simulink model "StraightACC_cs_old"  (R2016a)
settings: Solver=ode5  SolverMode=SingleTasking  StartTime=0.0  StopTime=10  FixedStep=1/1000  RelTol=1e-3
PreLoadFcn:
  | mbxruntime.callbacks.PreLoadFcn(bdroot);
PostLoadFcn:
  | mbxruntime.callbacks.PostLoadFcn(bdroot);
InitFcn:
  | mbxruntime.callbacks.InitFcn(bdroot);
StartFcn:
  | mbxruntime.callbacks.StartFcn(bdroot);
StopFcn:
  | mbxruntime.callbacks.StopFcn(bdroot);
model workspace (MAT data in the model file):
  mbox_table : struct (value not decoded)
  model_closed = 0
  sim_status = 0
values from neighbouring files (symbols this model uses):
  CCCDuration = 5    [PreScan_Runscript.m]
  V0 = CCCArray(2*CCCCasei-1)    [PreScan_Runscript.m]
  V1 = CCCArray(2*CCCCasei)    [PreScan_Runscript.m]
  VAccuracyIn = 0.8    [PreScan_Runscript.m]
  VDurationIn = 2    [PreScan_Runscript.m]
  VPIDIn = CCCArray(2*CCCCasei-1)    [PreScan_Runscript.m]
  VToleranceIn = 1    [PreScan_Runscript.m]
undefined symbols (not defined in the file or in its folder): ADASID, BMotor1, BMotor2, BrkDelayTime, DControlB, Delay1, Delay2, DiscIntNeverNeededParam, IControlB, JMotor1, JMotor2, PControlB, PreScanCarSimLoadFcn, ratioGearF, ratioGearR, TorqDelayTime, Tstep
undefined symbols (not defined in the file): WheelL0, WheelL1, WheelR0, WheelR1
libraries: simulink x13, simulink_extras x11, PreScanSimulinkLibrary x9, MyLib x3, Solver_SF x2, pil_lib x1, PreScanUsefulBlocks x1
(part 3 of 9)

== system StraightACC_cs_old/Roewe_550_S_Sedan_1/WheelDisplacement_Mux ==
  Steering Angle Front [rad] : Inport  Tag=inport/JointGroup  SampleTime=10/1000  BusOutputAsStruct=on
  Steering Angle Rear [rad] : Inport  Tag=inport/JointGroup  Port=2  SampleTime=10/1000  BusOutputAsStruct=on
  Rotation [rad] : Inport  Tag=inport/JointGroup  Port=3  SampleTime=10/1000  BusOutputAsStruct=on
  zDisp FL [m] : Inport  Tag=inport/JointGroup  Port=4  SampleTime=10/1000  BusOutputAsStruct=on
  zDisp FR [m] : Inport  Tag=inport/JointGroup  Port=5  SampleTime=10/1000  BusOutputAsStruct=on
  zDisp RL [m] : Inport  Tag=inport/JointGroup  Port=6  SampleTime=10/1000  BusOutputAsStruct=on
  zDisp RR [m] : Inport  Tag=inport/JointGroup  Port=7  SampleTime=10/1000  BusOutputAsStruct=on
  Ground_{1..12} (12 alike) : Ground
  WheelL0_Mux : Subsystem  Tag=mux/Joint  mask(PreScan Mux Block){DisplayName=WheelL0}
      mask prompts: DisplayName "Display Name"
      mask help:
      | This block simulates a generic joint used for generic models. This joint can be enabled/disabled from the GUI.
      |
      | For more information, please click Help.
      settings: DeleteFcn=PreScanBlockDeleteFcn;
      mask Help: eval('openHelp(254)')
  WheelL1_Mux : Subsystem  Tag=mux/Joint  mask(PreScan Mux Block){DisplayName=WheelL1}
      mask prompts: DisplayName "Display Name"
      mask help:
      | This block simulates a generic joint used for generic models. This joint can be enabled/disabled from the GUI.
      |
      | For more information, please click Help.
      settings: DeleteFcn=PreScanBlockDeleteFcn;
      mask Help: eval('openHelp(254)')
  WheelR0_Mux : Subsystem  Tag=mux/Joint  mask(PreScan Mux Block){DisplayName=WheelR0}
      mask prompts: DisplayName "Display Name"
      mask help:
      | This block simulates a generic joint used for generic models. This joint can be enabled/disabled from the GUI.
      |
      | For more information, please click Help.
      settings: DeleteFcn=PreScanBlockDeleteFcn;
      mask Help: eval('openHelp(254)')
  WheelR1_Mux : Subsystem  Tag=mux/Joint  mask(PreScan Mux Block){DisplayName=WheelR1}
      mask prompts: DisplayName "Display Name"
      mask help:
      | This block simulates a generic joint used for generic models. This joint can be enabled/disabled from the GUI.
      |
      | For more information, please click Help.
      settings: DeleteFcn=PreScanBlockDeleteFcn;
      mask Help: eval('openHelp(254)')
  WheelL0_Roewe_550_S_Sedan_1 : Outport  Tag=outport/JointActuator  OutDataTypeStr=Bus: PRESCAN_POSE_DATA  SampleTime=10/1000
  WheelL1_Roewe_550_S_Sedan_1 : Outport  Tag=outport/JointActuator  Port=2  OutDataTypeStr=Bus: PRESCAN_POSE_DATA  SampleTime=10/1000
  WheelR0_Roewe_550_S_Sedan_1 : Outport  Tag=outport/JointActuator  Port=3  OutDataTypeStr=Bus: PRESCAN_POSE_DATA  SampleTime=10/1000
  WheelR1_Roewe_550_S_Sedan_1 : Outport  Tag=outport/JointActuator  Port=4  OutDataTypeStr=Bus: PRESCAN_POSE_DATA  SampleTime=10/1000
  wires:
  WheelL0_Mux/1(Joint) -> WheelL0_Roewe_550_S_Sedan_1/1
  WheelL1_Mux/1(Joint) -> WheelL1_Roewe_550_S_Sedan_1/1
  WheelR0_Mux/1(Joint) -> WheelR0_Roewe_550_S_Sedan_1/1
  WheelR1_Mux/1(Joint) -> WheelR1_Roewe_550_S_Sedan_1/1
  Steering Angle Front [rad]/1 -> WheelR0_Mux/6(Yaw [rad]), WheelL0_Mux/6(Yaw [rad])
  Steering Angle Rear [rad]/1 -> WheelR1_Mux/6(Yaw [rad]), WheelL1_Mux/6(Yaw [rad])
  Rotation [rad]/1 -> WheelR0_Mux/5(Pitch [rad]), WheelL0_Mux/5(Pitch [rad]), WheelR1_Mux/5(Pitch [rad]), WheelL1_Mux/5(Pitch [rad])
  zDisp FL [m]/1 -> WheelL0_Mux/3(Z [m])
  zDisp FR [m]/1 -> WheelR0_Mux/3(Z [m])
  zDisp RL [m]/1 -> WheelL1_Mux/3(Z [m])
  zDisp RR [m]/1 -> WheelR1_Mux/3(Z [m])
  Ground_1/1 -> WheelL0_Mux/1(X [m])
  Ground_2/1 -> WheelL0_Mux/2(Y [m])
  Ground_3/1 -> WheelL0_Mux/4(Roll [rad])
  Ground_4/1 -> WheelL1_Mux/1(X [m])
  Ground_5/1 -> WheelL1_Mux/2(Y [m])
  Ground_6/1 -> WheelL1_Mux/4(Roll [rad])
  Ground_7/1 -> WheelR0_Mux/1(X [m])
  Ground_8/1 -> WheelR0_Mux/2(Y [m])
  Ground_9/1 -> WheelR0_Mux/4(Roll [rad])
  Ground_10/1 -> WheelR1_Mux/1(X [m])
  Ground_11/1 -> WheelR1_Mux/2(Y [m])
  Ground_12/1 -> WheelR1_Mux/4(Roll [rad])

== system StraightACC_cs_old/WheelL0_Roewe_550_S_Sedan_1/Actuator ==
  Joint : Inport
  Bus Selector : BusSelector  OutputSignals=POSITION,ORIENTATION
  visu_Rotate : Subsystem  mask(RPYActuator){UniqueID=UniqueID, Object3DID=Rotate_ObjectID3D, TimeStep=TimeStep}
      mask prompts: UniqueID "Auto-Assigned: Unique ID"; Object3DID "Auto-Assigned: Child 3D Object ID"; TimeStep "Auto-Assigned: Upload Period [s]"
      mask help: Applies angles update to selected child object
      mask Help:
      | Applies position update to selected child object
      | 
      | - UniqueID (double)   : Unique ID of the parent actor
      | - Object3DID (string) : Name of the child 3D object
      mask Display: port_label('input', 1, ['visu_Rotate_' Object3DID])
  visu_Translate : Subsystem  mask(PositionActuator){UniqueID=UniqueID, Object3DID=Translate_ObjectID3D, TimeStep=TimeStep}
      mask prompts: UniqueID "Auto-Assigned: Unique ID"; Object3DID "Auto-Assigned: Child 3D Object ID"; TimeStep "Auto-Assigned: Upload Period [s]"
      mask help: Applies position update to selected child object
      mask Help:
      | Applies position update to selected child object
      | 
      | - UniqueID (double)   : Unique ID of the parent actor
      | - Object3DID (string) : Name of the child 3D object
      mask Display: port_label('input', 1, ['visu_Translate_' Object3DID])
  wires:
  Bus Selector/2 -> visu_Rotate/1(In1)  "<ORIENTATION>"
  Bus Selector/1 -> visu_Translate/1(In1)  "<POSITION>"
  Joint/1 -> Bus Selector/1

== system StraightACC_cs_old/WheelL1_Roewe_550_S_Sedan_1/Actuator ==
  Joint : Inport
  Bus Selector : BusSelector  OutputSignals=POSITION,ORIENTATION
  visu_Rotate : Subsystem  mask(RPYActuator){UniqueID=UniqueID, Object3DID=Rotate_ObjectID3D, TimeStep=TimeStep}
      mask prompts: UniqueID "Auto-Assigned: Unique ID"; Object3DID "Auto-Assigned: Child 3D Object ID"; TimeStep "Auto-Assigned: Upload Period [s]"
      mask help: Applies angles update to selected child object
      mask Help:
      | Applies position update to selected child object
      | 
      | - UniqueID (double)   : Unique ID of the parent actor
      | - Object3DID (string) : Name of the child 3D object
      mask Display: port_label('input', 1, ['visu_Rotate_' Object3DID])
  visu_Translate : Subsystem  mask(PositionActuator){UniqueID=UniqueID, Object3DID=Translate_ObjectID3D, TimeStep=TimeStep}
      mask prompts: UniqueID "Auto-Assigned: Unique ID"; Object3DID "Auto-Assigned: Child 3D Object ID"; TimeStep "Auto-Assigned: Upload Period [s]"
      mask help: Applies position update to selected child object
      mask Help:
      | Applies position update to selected child object
      | 
      | - UniqueID (double)   : Unique ID of the parent actor
      | - Object3DID (string) : Name of the child 3D object
      mask Display: port_label('input', 1, ['visu_Translate_' Object3DID])
  wires:
  Bus Selector/2 -> visu_Rotate/1(In1)  "<ORIENTATION>"
  Bus Selector/1 -> visu_Translate/1(In1)  "<POSITION>"
  Joint/1 -> Bus Selector/1

== system StraightACC_cs_old/WheelR0_Roewe_550_S_Sedan_1/Actuator ==
  Joint : Inport
  Bus Selector : BusSelector  OutputSignals=POSITION,ORIENTATION
  visu_Rotate : Subsystem  mask(RPYActuator){UniqueID=UniqueID, Object3DID=Rotate_ObjectID3D, TimeStep=TimeStep}
      mask prompts: UniqueID "Auto-Assigned: Unique ID"; Object3DID "Auto-Assigned: Child 3D Object ID"; TimeStep "Auto-Assigned: Upload Period [s]"
      mask help: Applies angles update to selected child object
      mask Help:
      | Applies position update to selected child object
      | 
      | - UniqueID (double)   : Unique ID of the parent actor
      | - Object3DID (string) : Name of the child 3D object
      mask Display: port_label('input', 1, ['visu_Rotate_' Object3DID])
  visu_Translate : Subsystem  mask(PositionActuator){UniqueID=UniqueID, Object3DID=Translate_ObjectID3D, TimeStep=TimeStep}
      mask prompts: UniqueID "Auto-Assigned: Unique ID"; Object3DID "Auto-Assigned: Child 3D Object ID"; TimeStep "Auto-Assigned: Upload Period [s]"
      mask help: Applies position update to selected child object
      mask Help:
      | Applies position update to selected child object
      | 
      | - UniqueID (double)   : Unique ID of the parent actor
      | - Object3DID (string) : Name of the child 3D object
      mask Display: port_label('input', 1, ['visu_Translate_' Object3DID])
  wires:
  Bus Selector/2 -> visu_Rotate/1(In1)  "<ORIENTATION>"
  Bus Selector/1 -> visu_Translate/1(In1)  "<POSITION>"
  Joint/1 -> Bus Selector/1

== system StraightACC_cs_old/WheelR1_Roewe_550_S_Sedan_1/Actuator ==
  Joint : Inport
  Bus Selector : BusSelector  OutputSignals=POSITION,ORIENTATION
  visu_Rotate : Subsystem  mask(RPYActuator){UniqueID=UniqueID, Object3DID=Rotate_ObjectID3D, TimeStep=TimeStep}
      mask prompts: UniqueID "Auto-Assigned: Unique ID"; Object3DID "Auto-Assigned: Child 3D Object ID"; TimeStep "Auto-Assigned: Upload Period [s]"
      mask help: Applies angles update to selected child object
      mask Help:
      | Applies position update to selected child object
      | 
      | - UniqueID (double)   : Unique ID of the parent actor
      | - Object3DID (string) : Name of the child 3D object
      mask Display: port_label('input', 1, ['visu_Rotate_' Object3DID])
  visu_Translate : Subsystem  mask(PositionActuator){UniqueID=UniqueID, Object3DID=Translate_ObjectID3D, TimeStep=TimeStep}
      mask prompts: UniqueID "Auto-Assigned: Unique ID"; Object3DID "Auto-Assigned: Child 3D Object ID"; TimeStep "Auto-Assigned: Upload Period [s]"
      mask help: Applies position update to selected child object
      mask Help:
      | Applies position update to selected child object
      | 
      | - UniqueID (double)   : Unique ID of the parent actor
      | - Object3DID (string) : Name of the child 3D object
      mask Display: port_label('input', 1, ['visu_Translate_' Object3DID])
  wires:
  Bus Selector/2 -> visu_Rotate/1(In1)  "<ORIENTATION>"
  Bus Selector/1 -> visu_Translate/1(In1)  "<POSITION>"
  Joint/1 -> Bus Selector/1

== system StraightACC_cs_old/Audi_A8_Sedan_1/SELF_Demux/compas converter ==
  rotz [rad] : Inport
  cart2compas : Subsystem
  rad2deg : Gain  Gain=180/pi
  heading [deg] : Outport
  wires:
  rad2deg/1 -> cart2compas/1(Angle [deg])
  rotz [rad]/1 -> rad2deg/1
  cart2compas/1(heading [deg]) -> heading [deg]/1

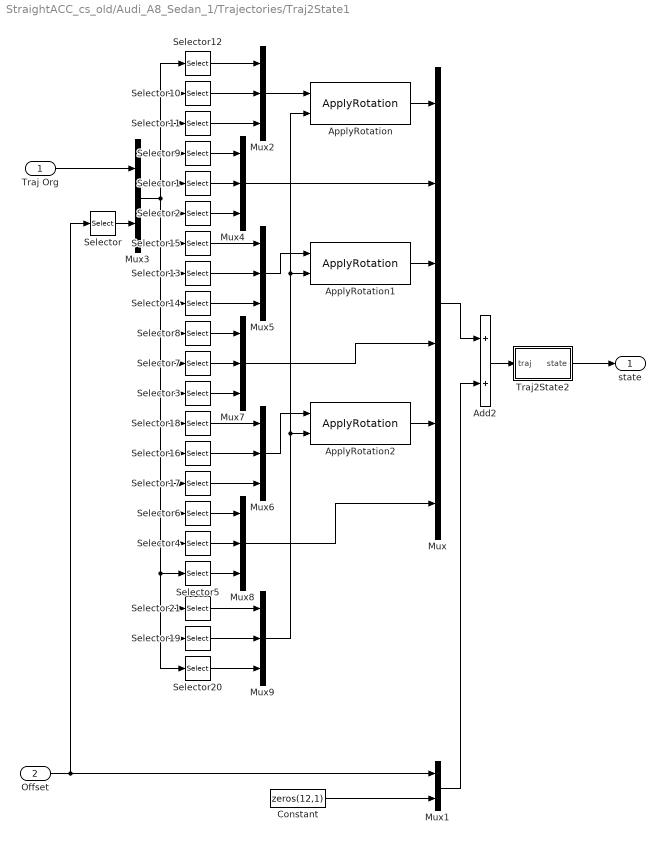
== system StraightACC_cs_old/Audi_A8_Sedan_1/Trajectories/Traj2State1 ==
  Traj Org : Inport
  Offset : Inport  Port=2
  Add2 : Sum
  ApplyRotation : PreScanSimulinkLibrary/ApplyRotation
  ApplyRotation1 : PreScanSimulinkLibrary/ApplyRotation
  ApplyRotation2 : PreScanSimulinkLibrary/ApplyRotation
  Constant : Constant  Value=zeros(12,1)
  Mux : Mux  Inputs=6
  Mux1 : Mux  Inputs=2
  Mux{2,4..9} (7 alike) : Mux  Inputs=3
  Mux3 : Mux  Inputs=2
  Selector : Selector  InputPortWidth=6  IndexOptions=Index vector (dialog)  Indices=[4 5 6]  OutputSizes=1
  Selector1 : Selector  InputPortWidth=21  IndexOptions=Index vector (dialog)  Indices=[5]  OutputSizes=1
  Selector10 : Selector  InputPortWidth=21  IndexOptions=Index vector (dialog)  Indices=[2]  OutputSizes=1
  Selector11 : Selector  InputPortWidth=21  IndexOptions=Index vector (dialog)  Indices=[3]  OutputSizes=1
  Selector12 : Selector  InputPortWidth=21  IndexOptions=Index vector (dialog)  Indices=[1]  OutputSizes=1
  Selector13 : Selector  InputPortWidth=21  IndexOptions=Index vector (dialog)  Indices=[8]  OutputSizes=1
  Selector14 : Selector  InputPortWidth=21  IndexOptions=Index vector (dialog)  Indices=[9]  OutputSizes=1
  Selector15 : Selector  InputPortWidth=21  IndexOptions=Index vector (dialog)  Indices=[7]  OutputSizes=1
  Selector16 : Selector  InputPortWidth=21  IndexOptions=Index vector (dialog)  Indices=[14]  OutputSizes=1
  Selector17 : Selector  InputPortWidth=21  IndexOptions=Index vector (dialog)  Indices=[15]  OutputSizes=1
  Selector18 : Selector  InputPortWidth=21  IndexOptions=Index vector (dialog)  Indices=[13]  OutputSizes=1
  Selector19 : Selector  InputPortWidth=21  IndexOptions=Index vector (dialog)  Indices=[20]  OutputSizes=1
  Selector2 : Selector  InputPortWidth=21  IndexOptions=Index vector (dialog)  Indices=[6]  OutputSizes=1
  Selector20 : Selector  InputPortWidth=21  IndexOptions=Index vector (dialog)  Indices=[21]  OutputSizes=1
  Selector21 : Selector  InputPortWidth=21  IndexOptions=Index vector (dialog)  Indices=[19]  OutputSizes=1
  Selector3 : Selector  InputPortWidth=21  IndexOptions=Index vector (dialog)  Indices=[12]  OutputSizes=1
  Selector4 : Selector  InputPortWidth=21  IndexOptions=Index vector (dialog)  Indices=[17]  OutputSizes=1
  Selector5 : Selector  InputPortWidth=21  IndexOptions=Index vector (dialog)  Indices=[18]  OutputSizes=1
  Selector6 : Selector  InputPortWidth=21  IndexOptions=Index vector (dialog)  Indices=[16]  OutputSizes=1
  Selector7 : Selector  InputPortWidth=21  IndexOptions=Index vector (dialog)  Indices=[11]  OutputSizes=1
  Selector8 : Selector  InputPortWidth=21  IndexOptions=Index vector (dialog)  Indices=[10]  OutputSizes=1
  Selector9 : Selector  InputPortWidth=21  IndexOptions=Index vector (dialog)  Indices=[4]  OutputSizes=1
  Traj2State2 : Subsystem
  state : Outport
  wires:
  Mux9/1 -> ApplyRotation2/2, ApplyRotation1/2, ApplyRotation/2
  Selector20/1 -> Mux9/3
  Selector19/1 -> Mux9/2
  Selector21/1 -> Mux9/1
  Selector5/1 -> Mux8/3
  Selector4/1 -> Mux8/2
  Selector6/1 -> Mux8/1
  Mux8/1 -> Mux/6
  Mux6/1 -> ApplyRotation2/1
  Mux7/1 -> Mux/4
  ApplyRotation2/1 -> Mux/5
  Selector3/1 -> Mux7/3
  Selector7/1 -> Mux7/2
  Selector8/1 -> Mux7/1
  Mux4/1 -> Mux/2
  Mux5/1 -> ApplyRotation1/1
  ApplyRotation1/1 -> Mux/3
  Mux2/1 -> ApplyRotation/1
  ApplyRotation/1 -> Mux/1
  Selector2/1 -> Mux4/3
  Selector1/1 -> Mux4/2
  Selector9/1 -> Mux4/1
  Selector17/1 -> Mux6/3
  Selector16/1 -> Mux6/2
  Selector18/1 -> Mux6/1
  Selector14/1 -> Mux5/3
  Selector13/1 -> Mux5/2
  Selector15/1 -> Mux5/1
  Selector11/1 -> Mux2/3
  Selector10/1 -> Mux2/2
  Selector12/1 -> Mux2/1
  Mux3/1 -> Selector8/1, Selector7/1, Selector3/1, Selector18/1, Selector16/1, Selector17/1, Selector6/1, Selector20/1, Selector19/1, Selector21/1, Selector5/1, Selector4/1, Selector14/1, Selector13/1, Selector15/1, Selector2/1, Selector1/1, Selector9/1, Selector12/1, Selector10/1, Selector11/1
  Mux1/1 -> Add2/2
  Constant/1 -> Mux1/2
  Add2/1 -> Traj2State2/1(traj)
  Selector/1 -> Mux3/2
  Traj Org/1 -> Mux3/1
  Offset/1 -> Mux1/1, Selector/1
  Mux/1 -> Add2/1
  Traj2State2/1(state) -> state/1

== system StraightACC_cs_old/Audi_A8_Sedan_1/Trajectories/TrajCoGOffset ==
  State In : Inport
  Add : Sum  Inputs=+-+
  Add1 : Sum
  ApplyRotation : PreScanSimulinkLibrary/ApplyRotation
  ApplyRotation1 : PreScanSimulinkLibrary/ApplyRotation
  CoG Offset : Constant  Value=[0 0 CoGOffsetZ]
  Degrees to Radians : simulink_extras/Transformations/Degrees to Radians
  Demux1 : Demux  Outputs=[3 3 3]
  Mux : Mux  Inputs=[3 3 3]
  Orientation : Constant  Value=[InitRoll InitPitch 0]
  State Out : Outport
  wires:
  State In/1 -> Demux1/1
  Demux1/1 -> Add/1
  Add/1 -> Mux/1
  Demux1/3 -> Mux/3, Add1/2
  Mux/1 -> State Out/1
  Demux1/2 -> Mux/2
  Orientation/1 -> Degrees to Radians/1
  ApplyRotation/1 -> Add/3
  ApplyRotation1/1 -> Add/2
  Add1/1 -> ApplyRotation/2
  CoG Offset/1 -> ApplyRotation1/1, ApplyRotation/1
  Degrees to Radians/1 -> Add1/1, ApplyRotation1/2

== system StraightACC_cs_old/Audi_A8_Sedan_1/Trajectories/Trajectory_1 ==
  From Workspace : FromWorkspace  VariableName=trajectory  SampleTime=TimeStep  OutputAfterFinalValue=Holding final value
  From Workspace1 : FromWorkspace  VariableName=trajectory  SampleTime=TimeStep  OutputAfterFinalValue=Setting to zero
  Mux : Mux  Inputs=2
  Selector1 : Selector  InputPortWidth=24  IndexOptions=Index vector (dialog)  Indices=[7:18]  OutputSizes=1
  Selector9 : Selector  InputPortWidth=24  IndexOptions=Index vector (dialog)  Indices=[1:6]  OutputSizes=1
  trajectory : Outport
  wires:
  From Workspace/1 -> Selector9/1
  From Workspace1/1 -> Selector1/1
  Mux/1 -> trajectory/1
  Selector9/1 -> Mux/1
  Selector1/1 -> Mux/2

== system StraightACC_cs_old/Roewe_550_S_Sedan_1/CarSim I//O/ACCAEB ==
  ACCAEBIn : Inport  OutDataTypeStr=Bus: AccAebInputs  BusOutputAsStruct=on
  ACCAEB_sfcn : pil_lib/PIL Block  SimulationMode=SIL  IsTopModelPIL=off  CodeDir=D:\Temp\SimCodeGen\Dest\ACCAEB_ert_rtw  ConfigName=Software-in-the-Loop (SIL)
  __InputSSForSFun__ : Subsystem
  __OutputSSForSFun__ : Subsystem
  ACCAEBOut : Outport
  wires:
  ACCAEBIn/1 -> __InputSSForSFun__/1(ACCAEBIn)
  __InputSSForSFun__/1(__UniqueOutportName__1__) -> ACCAEB_sfcn/1
  ACCAEB_sfcn/1 -> __OutputSSForSFun__/1(__UniqueInportName__1__)
  ACCAEB_sfcn/2 -> __OutputSSForSFun__/2(__UniqueInportName__2__)
  ACCAEB_sfcn/3 -> __OutputSSForSFun__/3(__UniqueInportName__3__)
  ACCAEB_sfcn/4 -> __OutputSSForSFun__/4(__UniqueInportName__4__)
  ACCAEB_sfcn/5 -> __OutputSSForSFun__/5(__UniqueInportName__5__)
  ACCAEB_sfcn/6 -> __OutputSSForSFun__/6(__UniqueInportName__6__)
  ACCAEB_sfcn/7 -> __OutputSSForSFun__/7(__UniqueInportName__7__)
  ACCAEB_sfcn/8 -> __OutputSSForSFun__/8(__UniqueInportName__8__)
  ACCAEB_sfcn/9 -> __OutputSSForSFun__/9(__UniqueInportName__9__)
  ACCAEB_sfcn/10 -> __OutputSSForSFun__/10(__UniqueInportName__10__)
  ACCAEB_sfcn/11 -> __OutputSSForSFun__/11(__UniqueInportName__11__)
  ACCAEB_sfcn/12 -> __OutputSSForSFun__/12(__UniqueInportName__12__)
  ACCAEB_sfcn/13 -> __OutputSSForSFun__/13(__UniqueInportName__13__)
  ACCAEB_sfcn/14 -> __OutputSSForSFun__/14(__UniqueInportName__14__)
  ACCAEB_sfcn/15 -> __OutputSSForSFun__/15(__UniqueInportName__15__)
  ACCAEB_sfcn/16 -> __OutputSSForSFun__/16(__UniqueInportName__16__)
  ACCAEB_sfcn/17 -> __OutputSSForSFun__/17(__UniqueInportName__17__)
  ACCAEB_sfcn/18 -> __OutputSSForSFun__/18(__UniqueInportName__18__)
  ACCAEB_sfcn/19 -> __OutputSSForSFun__/19(__UniqueInportName__19__)
  ACCAEB_sfcn/20 -> __OutputSSForSFun__/20(__UniqueInportName__20__)
  ACCAEB_sfcn/21 -> __OutputSSForSFun__/21(__UniqueInportName__21__)
  ACCAEB_sfcn/22 -> __OutputSSForSFun__/22(__UniqueInportName__22__)
  ACCAEB_sfcn/23 -> __OutputSSForSFun__/23(__UniqueInportName__23__)
  ACCAEB_sfcn/24 -> __OutputSSForSFun__/24(__UniqueInportName__24__)
  ACCAEB_sfcn/25 -> __OutputSSForSFun__/25(__UniqueInportName__25__)
  ACCAEB_sfcn/26 -> __OutputSSForSFun__/26(__UniqueInportName__26__)
  ACCAEB_sfcn/27 -> __OutputSSForSFun__/27(__UniqueInportName__27__)
  ACCAEB_sfcn/28 -> __OutputSSForSFun__/28(__UniqueInportName__28__)
  ACCAEB_sfcn/29 -> __OutputSSForSFun__/29(__UniqueInportName__29__)
  ACCAEB_sfcn/30 -> __OutputSSForSFun__/30(__UniqueInportName__30__)
  ACCAEB_sfcn/31 -> __OutputSSForSFun__/31(__UniqueInportName__31__)
  ACCAEB_sfcn/32 -> __OutputSSForSFun__/32(__UniqueInportName__32__)
  ACCAEB_sfcn/33 -> __OutputSSForSFun__/33(__UniqueInportName__33__)
  ACCAEB_sfcn/34 -> __OutputSSForSFun__/34(__UniqueInportName__34__)
  ACCAEB_sfcn/35 -> __OutputSSForSFun__/35(__UniqueInportName__35__)
  ACCAEB_sfcn/36 -> __OutputSSForSFun__/36(__UniqueInportName__36__)
  ACCAEB_sfcn/37 -> __OutputSSForSFun__/37(__UniqueInportName__37__)
  ACCAEB_sfcn/38 -> __OutputSSForSFun__/38(__UniqueInportName__38__)
  ACCAEB_sfcn/39 -> __OutputSSForSFun__/39(__UniqueInportName__39__)
  ACCAEB_sfcn/40 -> __OutputSSForSFun__/40(__UniqueInportName__40__)
  ACCAEB_sfcn/41 -> __OutputSSForSFun__/41(__UniqueInportName__41__)
  ACCAEB_sfcn/42 -> __OutputSSForSFun__/42(__UniqueInportName__42__)
  ACCAEB_sfcn/43 -> __OutputSSForSFun__/43(__UniqueInportName__43__)
  ACCAEB_sfcn/44 -> __OutputSSForSFun__/44(__UniqueInportName__44__)
  ACCAEB_sfcn/45 -> __OutputSSForSFun__/45(__UniqueInportName__45__)
  ACCAEB_sfcn/46 -> __OutputSSForSFun__/46(__UniqueInportName__46__)
  ACCAEB_sfcn/47 -> __OutputSSForSFun__/47(__UniqueInportName__47__)
  ACCAEB_sfcn/48 -> __OutputSSForSFun__/48(__UniqueInportName__48__)
  ACCAEB_sfcn/49 -> __OutputSSForSFun__/49(__UniqueInportName__49__)
  ACCAEB_sfcn/50 -> __OutputSSForSFun__/50(__UniqueInportName__50__)
  ACCAEB_sfcn/51 -> __OutputSSForSFun__/51(__UniqueInportName__51__)
  ACCAEB_sfcn/52 -> __OutputSSForSFun__/52(__UniqueInportName__52__)
  ACCAEB_sfcn/53 -> __OutputSSForSFun__/53(__UniqueInportName__53__)
  ACCAEB_sfcn/54 -> __OutputSSForSFun__/54(__UniqueInportName__54__)
  ACCAEB_sfcn/55 -> __OutputSSForSFun__/55(__UniqueInportName__55__)
  ACCAEB_sfcn/56 -> __OutputSSForSFun__/56(__UniqueInportName__56__)
  ACCAEB_sfcn/57 -> __OutputSSForSFun__/57(__UniqueInportName__57__)
  ACCAEB_sfcn/58 -> __OutputSSForSFun__/58(__UniqueInportName__58__)
  ACCAEB_sfcn/59 -> __OutputSSForSFun__/59(__UniqueInportName__59__)
  ACCAEB_sfcn/60 -> __OutputSSForSFun__/60(__UniqueInportName__60__)
  ACCAEB_sfcn/61 -> __OutputSSForSFun__/61(__UniqueInportName__61__)
  ACCAEB_sfcn/62 -> __OutputSSForSFun__/62(__UniqueInportName__62__)
  ACCAEB_sfcn/63 -> __OutputSSForSFun__/63(__UniqueInportName__63__)
  ACCAEB_sfcn/64 -> __OutputSSForSFun__/64(__UniqueInportName__64__)
  ACCAEB_sfcn/65 -> __OutputSSForSFun__/65(__UniqueInportName__65__)
  ACCAEB_sfcn/66 -> __OutputSSForSFun__/66(__UniqueInportName__66__)
  ACCAEB_sfcn/67 -> __OutputSSForSFun__/67(__UniqueInportName__67__)
  ACCAEB_sfcn/68 -> __OutputSSForSFun__/68(__UniqueInportName__68__)
  ACCAEB_sfcn/69 -> __OutputSSForSFun__/69(__UniqueInportName__69__)
  ACCAEB_sfcn/70 -> __OutputSSForSFun__/70(__UniqueInportName__70__)
  ACCAEB_sfcn/71 -> __OutputSSForSFun__/71(__UniqueInportName__71__)
  ACCAEB_sfcn/72 -> __OutputSSForSFun__/72(__UniqueInportName__72__)
  ACCAEB_sfcn/73 -> __OutputSSForSFun__/73(__UniqueInportName__73__)
  ACCAEB_sfcn/74 -> __OutputSSForSFun__/74(__UniqueInportName__74__)
  ACCAEB_sfcn/75 -> __OutputSSForSFun__/75(__UniqueInportName__75__)
  ACCAEB_sfcn/76 -> __OutputSSForSFun__/76(__UniqueInportName__76__)
  ACCAEB_sfcn/77 -> __OutputSSForSFun__/77(__UniqueInportName__77__)
  ACCAEB_sfcn/78 -> __OutputSSForSFun__/78(__UniqueInportName__78__)
  ACCAEB_sfcn/79 -> __OutputSSForSFun__/79(__UniqueInportName__79__)
  ACCAEB_sfcn/80 -> __OutputSSForSFun__/80(__UniqueInportName__80__)
  ACCAEB_sfcn/81 -> __OutputSSForSFun__/81(__UniqueInportName__81__)
  ACCAEB_sfcn/82 -> __OutputSSForSFun__/82(__UniqueInportName__82__)
  ACCAEB_sfcn/83 -> __OutputSSForSFun__/83(__UniqueInportName__83__)
  ACCAEB_sfcn/84 -> __OutputSSForSFun__/84(__UniqueInportName__84__)
  ACCAEB_sfcn/85 -> __OutputSSForSFun__/85(__UniqueInportName__85__)
  ACCAEB_sfcn/86 -> __OutputSSForSFun__/86(__UniqueInportName__86__)
  ACCAEB_sfcn/87 -> __OutputSSForSFun__/87(__UniqueInportName__87__)
  ACCAEB_sfcn/88 -> __OutputSSForSFun__/88(__UniqueInportName__88__)
  ACCAEB_sfcn/89 -> __OutputSSForSFun__/89(__UniqueInportName__89__)
  ACCAEB_sfcn/90 -> __OutputSSForSFun__/90(__UniqueInportName__90__)
  ACCAEB_sfcn/91 -> __OutputSSForSFun__/91(__UniqueInportName__91__)
  ACCAEB_sfcn/92 -> __OutputSSForSFun__/92(__UniqueInportName__92__)
  ACCAEB_sfcn/93 -> __OutputSSForSFun__/93(__UniqueInportName__93__)
  ACCAEB_sfcn/94 -> __OutputSSForSFun__/94(__UniqueInportName__94__)
  ACCAEB_sfcn/95 -> __OutputSSForSFun__/95(__UniqueInportName__95__)
  ACCAEB_sfcn/96 -> __OutputSSForSFun__/96(__UniqueInportName__96__)
  ACCAEB_sfcn/97 -> __OutputSSForSFun__/97(__UniqueInportName__97__)
  ACCAEB_sfcn/98 -> __OutputSSForSFun__/98(__UniqueInportName__98__)
  __OutputSSForSFun__/1(ACCAEBOut) -> ACCAEBOut/1

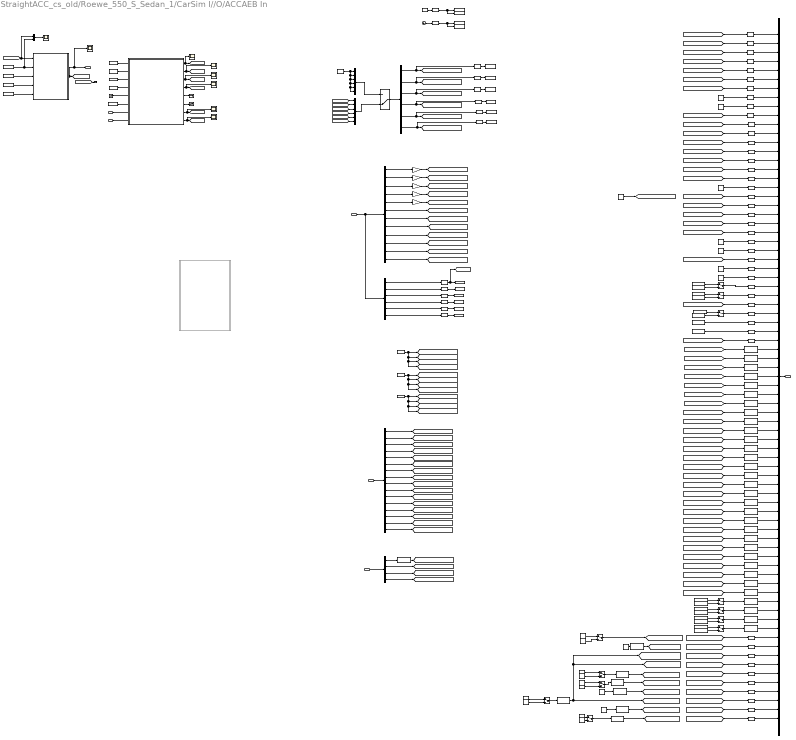
== system StraightACC_cs_old/Roewe_550_S_Sedan_1/CarSim I//O/ACCAEB In ==
  note: Here was constant 1, dont know why
  CarSimOut : Inport
  LanesInfo : Inport  Port=2
  FRadarOut : Inport  Port=3
  SetSpd : Inport  Port=4
  MemSpd : Inport  Port=5
  BrkPdlPos_H1HSC1_d1 : Constant  Value=0  OutDataTypeStr=double
  BrkPdlPos_H1HSC1_d2 : Constant  Value=0  OutDataTypeStr=uint8
  Bus Creator1 : BusCreator  Inputs=77
  Bus Selector : BusSelector  OutputSignals=Lane1C0,Lane1C1,Lane1C2,Lane1C3,Lane2C0,Lane2C1,Lane2C2,Lane2C3,Lane3C0,Lane3C1,Lane3C2,Lane3C3,Lane4C0,Lane4C1,Lane4C2,Lane4C3
  Bus Selector1 : BusSelector  OutputSignals=WhlGndVelRDrvn_H1HSC2_d[km/h] (signal 38),WhlGndVelLDrvn_H1HSC2_d[km/h] (signal 39),WhlGndVelRNonDrvn_H1HSC2_d[km/h] (signal 40),WhlGndVelLNonDrvn_H1HSC2_d[km/h] (signal 41),VSELongtAcc_H1HSC1_d[g] (signal 42),VehDynYawRate_H1HSC1_d[deg/s] (signal 43),EnSpdHSC1_d[rpm] (signal 36),SteeringWheelAngle[deg] (signal 34),StrgWhlAngGrd_HSC2_d[deg/s] (signal 44),EnToqActuExtdRngHSC1_d[N M] (signal 37),AccelEfctvPosHSC1_d (signal 46),AccelActuPosHSC1_d (signal 45)
  Bus Selector2 : BusSelector  OutputSignals=IDLockOn,Y_LockOn,X_LockOn,Vx_LockOn
  Bus Selector3 : BusSelector  OutputSignals=VehicleCoG_Vx[km/h] (signal 4),SteeringWheelAngle[deg] (signal 34),Ax_SM[g] (signal 54),Ay_SM[g] (signal 55),VehDynYawRate_H1HSC1_d[deg/s] (signal 43),StrgWhlAngGrd_HSC2_d[deg/s] (signal 44)
  CanclSW : Scope
  Chart : Stateflow chart  TreatAsAtomicUnit=on
  Clock1 : Clock
  Constant : Constant  Value=2
  Constant{1,5,13,93,102,104..105,107,110..111} (10 alike) : Constant  Value=0
  Constant{7,94,103,106,108..109,112..113} (8 alike) : Constant
  Constant15 : Constant  Value=VPIDIn
  Constant16 : Constant  Value=VToleranceIn
  Constant17 : Constant  Value=VAccuracyIn
  Constant18 : Constant  Value=VDurationIn
  Constant19 : Constant  Value=ADASID
  Constant2 : Constant  Value=95
  Constant20 : Constant  Value=V0
  Constant21 : Constant  Value=V1
  Constant3 : Constant  Value=1199
  Constant4 : Constant  Value=-848
  Constant6 : Constant  Value=CCCDuration
  DA_IN_DgrObjSyncCtr_u1 : Constant  Value=0  OutDataTypeStr=uint8
  DA_IN_DgrObjSyncCtr_u2 : Constant  Value=0  OutDataTypeStr=uint8
  DA_IN_DgrObjSyncCtr_u3 : Constant  Value=0  OutDataTypeStr=uint8
  Data Type Conversion{,1,4..8,10..12,23,28..29,31..32,45,58,66,73,86,89,115,120,124} (24 alike) : DataTypeConversion  OutDataTypeStr=uint8
  Data Type Conversion{2..3,13..22,24..27,30,35..40,84..85,92..94,116,126..129} (33 alike) : DataTypeConversion  OutDataTypeStr=double
  Data Type Conversion{9,87..88,90..91,117..119,121..123,125} (12 alike) : DataTypeConversion  OutDataTypeStr=single
  Data Type Conversion{33..34,80..83} (6 alike) : DataTypeConversion  OutDataTypeStr=boolean
  Data Type Conversion{46..48,55..57,60..65,67..72,74..79} (24 alike) : DataTypeConversion
  Demux : Demux  Outputs=6
  DrvrSbltAtcHSC1_u1 : Constant  OutDataTypeStr=uint8
  EPBAppcnStsHSC1_u1 : Constant  Value=0  OutDataTypeStr=uint8
  EnTypHSC2_u1 : Constant  OutDataTypeStr=uint8
  FntLatDist10 : Constant  Value=0  OutDataTypeStr=double
      settings: AttributesFormatString=%<OutDataTypeStr>
  FntLatDist11 : Constant  Value=13  OutDataTypeStr=double
      settings: AttributesFormatString=%<OutDataTypeStr>
  FntLatDist12 : Constant  Value=0  OutDataTypeStr=double
      settings: AttributesFormatString=%<OutDataTypeStr>
  FntLatDist7 : Constant  Value=3  OutDataTypeStr=double
      settings: AttributesFormatString=%<OutDataTypeStr>
  FntLatDist8 : Constant  Value=0  OutDataTypeStr=double
      settings: AttributesFormatString=%<OutDataTypeStr>
  FntLatDist9 : Constant  OutDataTypeStr=double
      settings: AttributesFormatString=%<OutDataTypeStr>
  Gain{,1..3} (4 alike) : Gain  Gain=1/3.6
  Gain4 : Gain  Gain=9.8
  Ground4 : Ground
  ID_LOCKON_u5 : Constant  Value=5  OutDataTypeStr=uint8
  ID_LOCKON_u6 : Constant  Value=0  OutDataTypeStr=uint8
  ID_LOCKON_u7 : Constant  Value=5  OutDataTypeStr=uint8
  ID_LOCKON_u9 : Constant  Value=0  OutDataTypeStr=uint8
  MATLAB Function : MATLAB Function  Commented=on  TreatAsAtomicUnit=on
  Manual Switch : ManualSwitch  CurrentSetting=0
  Manual Switch{56,60..70} (12 alike) : ManualSwitch
  Mux : Mux  Inputs=6
  Mux1 : Mux  Inputs=6
  Mux2 : Mux  Inputs=2
  OnSW : Scope
  RsmSW : Scope
  SetSW : Scope
  SpdDecSW : Scope
  SpdIncSW : Scope
  Steady? : Scope
  SysPwrMd_H1HSC1_u1 : Constant  Value=3  OutDataTypeStr=uint8
      settings: AttributesFormatString=%<DataType=%<OutDataTypeStr>>
  Terminator4 : Terminator
  Terminator5 : Terminator
  Terminator_1 : Terminator
  To Workspace : ToWorkspace  VariableName=SpdIncSw  SampleTime=-1
  To Workspace1 : ToWorkspace  VariableName=SpdDecSw  SampleTime=-1
  To Workspace10 : ToWorkspace  VariableName=Vx  SampleTime=-1
  To Workspace11 : ToWorkspace  VariableName=AVz  SampleTime=-1
  To Workspace12 : ToWorkspace  VariableName=Steer_SW  SampleTime=-1
  To Workspace13 : ToWorkspace  VariableName=StrAV_SW  SampleTime=-1
  To Workspace14 : ToWorkspace  VariableName=Time  SampleTime=-1
  To Workspace15 : ToWorkspace  VariableName=T_Stamp  SampleTime=-1
  To Workspace2 : ToWorkspace  VariableName=SetSw  SampleTime=-1
  To Workspace3 : ToWorkspace  VariableName=CanclSw  SampleTime=-1
  To Workspace4 : ToWorkspace  VariableName=RsmSw  SampleTime=-1
  To Workspace5 : ToWorkspace  VariableName=OnSw  SampleTime=-1
  To Workspace6 : ToWorkspace  VariableName=DisIncSw  SampleTime=-1
  To Workspace7 : ToWorkspace  VariableName=DisDecSw  SampleTime=-1
  To Workspace8 : ToWorkspace  VariableName=Ax  SampleTime=-1
  To Workspace9 : ToWorkspace  VariableName=Ay  SampleTime=-1
  TrEstdGear_HSC1_u1 : Constant  Value=4  OutDataTypeStr=uint8
  TrShftLvrPosHSC1_u1 : Constant  Value=4  OutDataTypeStr=uint8
  V Compare : Scope
  isSteady : Subsystem
  ACCAEBInput : Outport  OutDataTypeStr=Bus: AccAebInputs
  SteadyFlag : Outport  Port=2
  wires:
  LanesInfo/1 -> Bus Selector/1
  TrEstdGear_HSC1_u1/1 -> Data Type Conversion28/1  "TrEstdGear_HSC1_u8"
  [StrgWhlAngGrd_HSC2_d] -> Data Type Conversion24/1  "StrgWhlAngGrd_HSC2_d"
  [VELOCITY_LOCKON_d] -> Data Type Conversion14/1  "VELOCITY_LOCKON_d"
  [X_POSITION_LOCKON_d] -> Data Type Conversion19/1  "X_POSITION_LOCKON_d"
  [VehDynYawRate_H1HSC1_d] -> Data Type Conversion27/1
  [PtBrkPdlDscrtInptStsHSC1_u8] -> Data Type Conversion23/1  "PtBrkPdlDscrtInptStsHSC1_u8"
  BrkPdlPos_H1HSC1_d1/1 -> Data Type Conversion22/1  "BrkPdlPos_H1HSC1_d"
  TrShftLvrPosHSC1_u1/1 -> Data Type Conversion12/1  "TrShftLvrPosHSC1_u8"
  Bus Creator1/1 -> ACCAEBInput/1
  EnTypHSC2_u1/1 -> Data Type Conversion29/1  "EnTypHSC2_u8"
  DrvrSbltAtcHSC1_u1/1 -> Data Type Conversion31/1  "DrvrSbltAtcHSC1_u8"
  EPBAppcnStsHSC1_u1/1 -> Data Type Conversion32/1  "EPBAppcnStsHSC1_u8"
  SysPwrMd_H1HSC1_u1/1 -> Data Type Conversion11/1  "SysPwrMd_H1HSC1_u8"
  [VSELongtAcc_H1HSC1_d] -> Data Type Conversion21/1  "VSELongtAcc_H1HSC1_d"
  [StrgWhlAngHSC2_d] -> Data Type Conversion25/1  "StrgWhlAngHSC2_d"
  [WhlGndVelRDrvn_H1HSC2_d] -> Data Type Conversion15/1  "WhlGndVelRDrvn_H1HSC2_d"
  [WhlGndVelLDrvn_H1HSC2_d] -> Data Type Conversion16/1  "WhlGndVelLDrvn_H1HSC2_d"
  [WhlGndVelRNonDrvn_H1HSC2_d] -> Data Type Conversion17/1  "WhlGndVelRNonDrvn_H1HSC2_d"
  [WhlGndVelLNonDrvn_H1HSC2_d] -> Data Type Conversion18/1  "WhlGndVelLNonDrvn_H1HSC2_d"
  [EnSpdHSC1_d] -> Data Type Conversion30/1  "EnSpdHSC1_d"
  [Y_POSITION_LOCKON_d] -> Data Type Conversion20/1  "Y_POSITION_LOCKON_d"
  [CCSwStsSpdIncSwAHSC1_u8] -> Data Type Conversion4/1  "CCSwStsSpdIncSwAHSC1_u8"
  [CCSwStsSpdDecSwAHSC1_u8] -> Data Type Conversion5/1  "CCSwStsSpdDecSwAHSC1_u8"
  [CCSwStsSetSwAHSC1_u8] -> Data Type Conversion6/1  "CCSwStsSetSwAHSC1_u8"
  [CCSwStsRsmSwAHSC1_u8] -> Data Type Conversion7/1  "CCSwStsRsmSwAHSC1_u8"
  [CCSwStsOnSwAHSC1_u8] -> Data Type Conversion8/1  "CCSwStsOnSwAHSC1_u8"
  [CCSwStsCanclSwAHSC1_u8] -> Data Type Conversion10/1  "CCSwStsCanclSwAHSC1_u8"
  [AccelActuPosHSC1_d] -> Data Type Conversion26/1  "AccelActuPosHSC1_d"
  [EnToqActuExtdRngHSC1_d] -> Data Type Conversion35/1  "EnToqActuExtdRngHSC1_d"
  Manual Switch56/1 -> Data Type Conversion36/1
  Constant94/1 -> Manual Switch56/2
  Constant93/1 -> Manual Switch56/1
  Data Type Conversion36/1 -> Bus Creator1/32  "EnToqDrvrReqdExtdRngHSC1_d"
  Data Type Conversion37/1 -> Bus Creator1/33  "EnToqMinExtdRngHSC1_d"
  Data Type Conversion38/1 -> Bus Creator1/34  "EnToqMaxExtdRngHSC1_d"
  [AccelEfctvPosHSC1_d] -> Data Type Conversion39/1  "AccelEfctvPosHSC1_d"
  Data Type Conversion45/1 -> Bus Creator1/36  "Lane0_Lane_Mark_Quality"
  Data Type Conversion46/1 -> Bus Creator1/37  "Lane0_Lane_View_Range_Start"
  Data Type Conversion47/1 -> Bus Creator1/38  "Lane0_Lane_View_Range_End"
  Data Type Conversion48/1 -> Bus Creator1/39  "Lane0_C0_Lane_Position"
  Data Type Conversion55/1 -> Bus Creator1/40  "Lane0_C1_Heading_Angle"
  Data Type Conversion56/1 -> Bus Creator1/41  "Lane0_C2_Lane_Curvature"
  Data Type Conversion57/1 -> Bus Creator1/42  "Lane0_C3_Lane_Curvature_Driv"
  Data Type Conversion58/1 -> Bus Creator1/43  "Lane1_Lane_Mark_Quality"
  Data Type Conversion60/1 -> Bus Creator1/44  "Lane1_Lane_View_Range_Start"
  Data Type Conversion61/1 -> Bus Creator1/45  "Lane1_Lane_View_Range_End"
  Data Type Conversion62/1 -> Bus Creator1/46  "Lane1_C0_Lane_Position"
  Data Type Conversion63/1 -> Bus Creator1/47  "Lane1_C1_Heading_Angle"
  Data Type Conversion64/1 -> Bus Creator1/48  "Lane1_C2_Lane_Curvature"
  Data Type Conversion65/1 -> Bus Creator1/49  "Lane1_C3_Lane_Curvature_Driv"
  Data Type Conversion66/1 -> Bus Creator1/50  "Lane2_Lane_Mark_Quality"
  Data Type Conversion67/1 -> Bus Creator1/51  "Lane2_Lane_View_Range_Start"
  Data Type Conversion68/1 -> Bus Creator1/52  "Lane2_Lane_View_Range_End"
  Data Type Conversion69/1 -> Bus Creator1/53  "Lane2_C0_Lane_Position"
  Data Type Conversion70/1 -> Bus Creator1/54  "Lane2_C1_Heading_Angle"
  Data Type Conversion71/1 -> Bus Creator1/55  "Lane2_C2_Lane_Curvature"
  Data Type Conversion72/1 -> Bus Creator1/56  "Lane2_C3_Lane_Curvature_Driv"
  Manual Switch60/1 -> Data Type Conversion80/1
  Constant103/1 -> Manual Switch60/2
  Constant102/1 -> Manual Switch60/1
  Manual Switch63/1 -> Data Type Conversion81/1
  Constant109/1 -> Manual Switch63/2
  Constant104/1 -> Manual Switch63/1
  Manual Switch61/1 -> Data Type Conversion82/1
  Constant106/1 -> Manual Switch61/2
  Constant105/1 -> Manual Switch61/1
  Manual Switch62/1 -> Data Type Conversion83/1
  Constant108/1 -> Manual Switch62/2
  Constant107/1 -> Manual Switch62/1
  Data Type Conversion78/1 -> Bus Creator1/62  "Lane3_C2_Lane_Curvature"
  Data Type Conversion83/1 -> Bus Creator1/67  "MainBeamLghtOnHSC1"
  Data Type Conversion79/1 -> Bus Creator1/63  "Lane3_C3_Lane_Curvature_Driv"
  Data Type Conversion81/1 -> Bus Creator1/65  "FrtFogLghtOnHSC1"
  Data Type Conversion77/1 -> Bus Creator1/61  "Lane3_C1_Heading_Angle"
  Data Type Conversion82/1 -> Bus Creator1/66  "DipdBeamLghtOnHSC1"
  Data Type Conversion80/1 -> Bus Creator1/64  "RrFogLghtOnHSC1_b"
  Data Type Conversion75/1 -> Bus Creator1/59  "Lane3_Lane_View_Range_End"
  Data Type Conversion76/1 -> Bus Creator1/60  "Lane3_C0_Lane_Position"
  Data Type Conversion73/1 -> Bus Creator1/57  "Lane3_Lane_Mark_Quality"
  Data Type Conversion74/1 -> Bus Creator1/58  "Lane3_Lane_View_Range_Start"
  Manual Switch65/1 -> Data Type Conversion33/1
  Constant113/1 -> Manual Switch65/2
  Constant110/1 -> Manual Switch65/1
  Data Type Conversion33/1 -> Bus Creator1/29  "RDircnIOHSC1_b"
  Manual Switch64/1 -> Data Type Conversion34/1
  Constant112/1 -> Manual Switch64/2
  Constant111/1 -> Manual Switch64/1
  Data Type Conversion34/1 -> Bus Creator1/30  "LDircnIOHSC1_b"
  [DA_IN_indx_RCARrTgtID_u8] -> Data Type Conversion115/1  "DA_IN_indx_RCARrTgtID_u8"
  [DA_IN_v_RMRltVehSpd_sg] -> Data Type Conversion117/1  "DA_IN_v_RMRltVehSpd_sg"
  [DA_IN_d_RMRdrLongtDist_sg] -> Data Type Conversion119/1  "DA_IN_d_RMRdrLongtDist_sg"
  [DA_IN_DgrObjId_u8] -> Data Type Conversion120/1  "DA_IN_DgrObjId_u8"
  [DA_IN_DgrObjLatRltvDist_sg] -> Data Type Conversion121/1  "DA_IN_DgrObjLatRltvDist_sg"
  [DA_IN_DgrObjLatRltvSpd_sg] -> Data Type Conversion122/1  "DA_IN_DgrObjLatRltvSpd_sg"
  [DA_IN_DgrObjLongtRltvSpd_sg] -> Data Type Conversion125/1  "DA_IN_DgrObjLongtRltvSpd_sg"
  [DA_IN_DgrObjLongtRltvDist_sg] -> Data Type Conversion123/1  "DA_IN_DgrObjLongtRltvDist_sg"
  [DA_IN_DgrObjSyncCtr_u8] -> Data Type Conversion124/1  "DA_IN_DgrObjSyncCtr_u8"
  [DA_IN_d_RMRdrLatDist_sg] -> Data Type Conversion118/1  "DA_IN_d_RMRdrLatDist_sg"
  ID_LOCKON_u5/1 -> Manual Switch66/1
  ID_LOCKON_u6/1 -> Manual Switch66/2
  Manual Switch66/1 -> Data Type Conversion86/1
  ID_LOCKON_u7/1 -> Manual Switch67/1
  ID_LOCKON_u9/1 -> Manual Switch67/2
  Manual Switch67/1 -> [DA_IN_indx_RCARrTgtID_u8]
  Data Type Conversion86/1 -> [DA_IN_DgrObjId_u8]
  FntLatDist11/1 -> Manual Switch68/1
  FntLatDist12/1 -> Manual Switch68/2
  Manual Switch68/1 -> Data Type Conversion88/1
  FntLatDist9/1 -> Manual Switch69/1
  FntLatDist10/1 -> Manual Switch69/2
  Manual Switch69/1 -> Data Type Conversion87/1
  FntLatDist7/1 -> Manual Switch70/1
  FntLatDist8/1 -> Manual Switch70/2
  Manual Switch70/1 -> Data Type Conversion90/1
  DA_IN_DgrObjSyncCtr_u3/1 -> Data Type Conversion91/1
  Data Type Conversion87/1 -> [DA_IN_DgrObjLatRltvDist_sg]
  Data Type Conversion88/1 -> [DA_IN_DgrObjLongtRltvDist_sg], [DA_IN_d_RMRdrLongtDist_sg], [DA_IN_d_RMRdrLatDist_sg]
  Data Type Conversion89/1 -> [DA_IN_DgrObjSyncCtr_u8]
  Data Type Conversion90/1 -> [DA_IN_DgrObjLongtRltvSpd_sg]
  Data Type Conversion91/1 -> [DA_IN_v_RMRltVehSpd_sg]
  [ID_LOCKON_u8] -> Data Type Conversion1/1  "ID_LOCKON_u8"
  [Lane2_Lane_Mark_Quality] -> Data Type Conversion58/1
  [Lane2_Lane_View_Range_Start] -> Data Type Conversion60/1
  [Lane2_Lane_View_Range_End] -> Data Type Conversion61/1
  [Lane2_C0_Lane_Position] -> Data Type Conversion62/1
  [Lane2_C1_Heading_Angle] -> Data Type Conversion63/1
  [Lane2_C2_Lane_Curvature] -> Data Type Conversion64/1
  [Lane2_C3_Lane_Curvature_Driv] -> Data Type Conversion65/1
  [Lane4_Lane_Mark_Quality] -> Data Type Conversion73/1
  [Lane4_Lane_View_Range_Start] -> Data Type Conversion74/1
  [Lane4_Lane_View_Range_End] -> Data Type Conversion75/1
  [Lane4_C0_Lane_Position] -> Data Type Conversion76/1
  [Lane4_C1_Heading_Angle] -> Data Type Conversion77/1
  [Lane4_C2_Lane_Curvature] -> Data Type Conversion78/1
  [Lane4_C3_Lane_Curvature_Driv] -> Data Type Conversion79/1
  DA_IN_DgrObjSyncCtr_u1/1 -> Data Type Conversion9/1
  Data Type Conversion9/1 -> [DA_IN_DgrObjLatRltvSpd_sg]
  DA_IN_DgrObjSyncCtr_u2/1 -> Data Type Conversion89/1
  CarSimOut/1 -> Bus Selector3/1, Bus Selector1/1
  FRadarOut/1 -> Bus Selector2/1
  Bus Selector2/1 -> Data Type Conversion/1  "<IDLockOn>"
  Bus Selector2/4 -> [VELOCITY_LOCKON_d]  "<Vx_LockOn>"
  Bus Selector2/3 -> [X_POSITION_LOCKON_d]  "<X_LockOn>"
  Bus Selector2/2 -> [Y_POSITION_LOCKON_d]  "<Y_LockOn>"
  Constant/1 -> [Lane4_Lane_Mark_Quality], [Lane3_Lane_Mark_Quality], [Lane2_Lane_Mark_Quality], [Lane1_Lane_Mark_Quality]
  Constant1/1 -> [Lane4_Lane_View_Range_Start], [Lane3_Lane_View_Range_Start], [Lane2_Lane_View_Range_Start], [Lane1_Lane_View_Range_Start]
  Constant2/1 -> [Lane4_Lane_View_Range_End], [Lane3_Lane_View_Range_End], [Lane2_Lane_View_Range_End], [Lane1_Lane_View_Range_End]
  Bus Selector1/1 -> Gain/1  "<WhlGndVelRDrvn_H1HSC2_d[km/h] (signal 38)>"
  Bus Selector1/2 -> Gain1/1  "<WhlGndVelLDrvn_H1HSC2_d[km/h] (signal 39)>"
  Bus Selector1/3 -> Gain2/1  "<WhlGndVelRNonDrvn_H1HSC2_d[km/h] (signal 40)>"
  Bus Selector1/4 -> Gain3/1  "<WhlGndVelLNonDrvn_H1HSC2_d[km/h] (signal 41)>"
  Bus Selector1/5 -> Gain4/1  "<VSELongtAcc_H1HSC1_d[g] (signal 42)>"
  Bus Selector1/6 -> [VehDynYawRate_H1HSC1_d]  "<VehDynYawRate_H1HSC1_d[deg/s] (signal 43)>"
  Bus Selector1/7 -> [EnSpdHSC1_d]  "<EnSpdHSC1_d[rpm] (signal 36)>"
  Bus Selector1/8 -> [StrgWhlAngHSC2_d]  "<SteeringWheelAngle[deg] (signal 34)>"
  Bus Selector1/9 -> [StrgWhlAngGrd_HSC2_d]  "<StrgWhlAngGrd_HSC2_d[deg/s] (signal 44)>"
  Gain/1 -> [WhlGndVelRDrvn_H1HSC2_d]
  Gain1/1 -> [WhlGndVelLDrvn_H1HSC2_d]
  Gain2/1 -> [WhlGndVelRNonDrvn_H1HSC2_d]
  Gain3/1 -> [WhlGndVelLNonDrvn_H1HSC2_d]
  Gain4/1 -> [VSELongtAcc_H1HSC1_d]
  Constant3/1 -> Data Type Conversion38/1
  Constant4/1 -> Data Type Conversion37/1
  Bus Selector1/12 -> [AccelActuPosHSC1_d]  "<AccelActuPosHSC1_d (signal 45)>"
  Bus Selector1/11 -> [AccelEfctvPosHSC1_d]  "<AccelEfctvPosHSC1_d (signal 46)>"
  Bus Selector1/10 -> [EnToqActuExtdRngHSC1_d]  "<EnToqActuExtdRngHSC1_d[N M] (signal 37)>"
  BrkPdlPos_H1HSC1_d2/1 -> [PtBrkPdlDscrtInptStsHSC1_u8]
  Demux/6 -> [CCSwStsCanclSwAHSC1_u8], Data Type Conversion94/1
  Demux/3 -> Data Type Conversion2/1, [CCSwStsSpdIncSwAHSC1_u8]
  Demux/4 -> Data Type Conversion84/1, [CCSwStsSpdDecSwAHSC1_u8]
  Demux/5 -> [CCSwStsRsmSwAHSC1_u8], Data Type Conversion92/1
  Data Type Conversion/1 -> [ID_LOCKON_u8]
  Data Type Conversion4/1 -> Bus Creator1/2  "CCSwStsSpdIncSwAHSC1_u8"
  Data Type Conversion5/1 -> Bus Creator1/3  "CCSwStsSpdDecSwAHSC1_u8"
  Data Type Conversion6/1 -> Bus Creator1/4  "CCSwStsSetSwAHSC1_u8"
  Data Type Conversion7/1 -> Bus Creator1/5  "CCSwStsRsmSwAHSC1_u8"
  Data Type Conversion8/1 -> Bus Creator1/6  "CCSwStsOnSwAHSC1_u8"
  Data Type Conversion10/1 -> Bus Creator1/7  "CCSwStsCanclSwAHSC1_u8"
  Data Type Conversion11/1 -> Bus Creator1/8  "SysPwrMd_H1HSC1_u8"
  Data Type Conversion12/1 -> Bus Creator1/9  "TrShftLvrPosHSC1_u8"
  Data Type Conversion14/1 -> Bus Creator1/10  "VELOCITY_LOCKON_d"
  Data Type Conversion15/1 -> Bus Creator1/11  "WhlGndVelRDrvn_H1HSC2_d"
  Data Type Conversion16/1 -> Bus Creator1/12  "WhlGndVelLDrvn_H1HSC2_d"
  Data Type Conversion17/1 -> Bus Creator1/13  "WhlGndVelRNonDrvn_H1HSC2_d"
  Data Type Conversion18/1 -> Bus Creator1/14  "WhlGndVelLNonDrvn_H1HSC2_d"
  Data Type Conversion19/1 -> Bus Creator1/15  "X_POSITION_LOCKON_d"
  Data Type Conversion20/1 -> Bus Creator1/16  "Y_POSITION_LOCKON_d"
  Data Type Conversion1/1 -> Bus Creator1/1  "ID_LOCKON_u8"
  Data Type Conversion21/1 -> Bus Creator1/17  "VSELongtAcc_H1HSC1_d"
  Data Type Conversion22/1 -> Bus Creator1/18  "BrkPdlPos_H1HSC1_d"
  Data Type Conversion23/1 -> Bus Creator1/19  "PtBrkPdlDscrtInptStsHSC1_u8"
  Data Type Conversion24/1 -> Bus Creator1/20  "StrgWhlAngGrd_HSC2_d"
  Data Type Conversion25/1 -> Bus Creator1/21  "StrgWhlAngHSC2_d"
  Data Type Conversion26/1 -> Bus Creator1/22  "AccelActuPosHSC1_d"
  Data Type Conversion27/1 -> Bus Creator1/23  "VehDynYawRate_H1HSC1_d"
  Data Type Conversion28/1 -> Bus Creator1/24  "TrEstdGear_HSC1_u8"
  Data Type Conversion29/1 -> Bus Creator1/25  "EnTypHSC2_u8"
  Data Type Conversion30/1 -> Bus Creator1/26  "EnSpdHSC1_d"
  Data Type Conversion31/1 -> Bus Creator1/27  "DrvrSbltAtcHSC1_u8"
  Data Type Conversion32/1 -> Bus Creator1/28  "EPBAppcnStsHSC1_u8"
  Data Type Conversion35/1 -> Bus Creator1/31  "EnToqActuExtdRngHSC1_d"
  Data Type Conversion39/1 -> Bus Creator1/35  "AccelEfctvPosHSC1_d"
  Data Type Conversion115/1 -> Bus Creator1/68  "DA_IN_indx_RCARrTgtID_u8"
  Data Type Conversion117/1 -> Bus Creator1/69  "DA_IN_v_RMRltVehSpd_sg"
  Data Type Conversion118/1 -> Bus Creator1/70  "DA_IN_d_RMRdrLatDist_sg"
  Data Type Conversion119/1 -> Bus Creator1/71  "DA_IN_d_RMRdrLongtDist_sg"
  Data Type Conversion120/1 -> Bus Creator1/72  "DA_IN_DgrObjId_u8"
  Data Type Conversion121/1 -> Bus Creator1/73  "DA_IN_DgrObjLatRltvDist_sg"
  Data Type Conversion122/1 -> Bus Creator1/74  "DA_IN_DgrObjLatRltvSpd_sg"
  Data Type Conversion123/1 -> Bus Creator1/75  "DA_IN_DgrObjLongtRltvDist_sg"
  Data Type Conversion124/1 -> Bus Creator1/76  "DA_IN_DgrObjSyncCtr_u8"
  Data Type Conversion125/1 -> Bus Creator1/77  "DA_IN_DgrObjLongtRltvSpd_sg"
  Demux/1 -> Data Type Conversion93/1, [CCSwStsOnSwAHSC1_u8]
  Constant13/1 -> Data Type Conversion3/1
  Data Type Conversion3/1 -> To Workspace7/1, To Workspace6/1
  Data Type Conversion129/1 -> To Workspace8/1
  Data Type Conversion127/1 -> To Workspace11/1
  Data Type Conversion116/1 -> To Workspace13/1
  Data Type Conversion13/1 -> To Workspace12/1
  Data Type Conversion126/1 -> [CarSimVx], To Workspace10/1
  Data Type Conversion128/1 -> To Workspace9/1
  Data Type Conversion40/1 -> To Workspace15/1, To Workspace14/1
  Clock1/1 -> Data Type Conversion40/1
  Data Type Conversion2/1 -> To Workspace/1
  Data Type Conversion84/1 -> To Workspace1/1
  Data Type Conversion85/1 -> To Workspace2/1
  Data Type Conversion92/1 -> To Workspace4/1
  Data Type Conversion93/1 -> To Workspace5/1
  Data Type Conversion94/1 -> To Workspace3/1
  Bus Selector3/1 -> Data Type Conversion126/1  "<VehicleCoG_Vx[km/h] (signal 4)>"
  Bus Selector3/2 -> Data Type Conversion13/1  "<SteeringWheelAngle[deg] (signal 34)>"
  Bus Selector3/3 -> Data Type Conversion129/1  "<Ax_SM[g] (signal 54)>"
  Bus Selector3/4 -> Data Type Conversion128/1  "<Ay_SM[g] (signal 55)>"
  Bus Selector3/5 -> Data Type Conversion127/1  "<VehDynYawRate_H1HSC1_d[deg/s] (signal 43)>"
  Bus Selector3/6 -> Data Type Conversion116/1  "<StrgWhlAngGrd_HSC2_d[deg/s] (signal 44)>"
  Chart/1(OnSW) -> OnSW/1, [OnSW]
  Chart/3(SpdIncSW) -> SpdIncSW/1, [SpdIncSW]
  Chart/4(SpdDecSW) -> SpdDecSW/1, [SpdDecSW]
  Chart/5(DisIncSW) -> Terminator4/1
  Chart/6(DisDecSW) -> Terminator5/1
  Chart/7(CanclSW) -> CanclSW/1, [CanclSW]
  Chart/8(RsmSW) -> RsmSW/1, [RsmSW]
  Chart/2(SetSW) -> SetSW/1, [SetSW]
  Constant19/1 -> Chart/1(ADASID)
  Constant20/1 -> Chart/3(V0)
  Constant21/1 -> Chart/4(V1)
  Ground4/1 -> Chart/5(Interval)
  [CarSimVx] -> Mux2/1, isSteady/1(Vx)
  isSteady/1(SteadyFlag) -> Steady?/1, SteadyFlag/1, [SteadyFlag]
  Constant15/1 -> Mux2/2, isSteady/2(VSet)
  Constant16/1 -> isSteady/3(VError)
  Constant17/1 -> isSteady/4(Accuracy)
  Constant18/1 -> isSteady/5(VDuration)
  Bus Selector/12 -> [Lane3_C3_Lane_Curvature_Driv]  "<Lane3C3>"
  Bus Selector/14 -> [Lane4_C1_Heading_Angle]  "<Lane4C1>"
  Bus Selector/10 -> [Lane3_C1_Heading_Angle]  "<Lane3C1>"
  Bus Selector/4 -> [Lane1_C3_Lane_Curvature_Driv]  "<Lane1C3>"
  Bus Selector/8 -> [Lane2_C3_Lane_Curvature_Driv]  "<Lane2C3>"
  Bus Selector/7 -> [Lane2_C2_Lane_Curvature]  "<Lane2C2>"
  Bus Selector/1 -> [Lane1_C0_Lane_Position]  "<Lane1C0>"
  Bus Selector/15 -> [Lane4_C2_Lane_Curvature]  "<Lane4C2>"
  Bus Selector/3 -> [Lane1_C2_Lane_Curvature]  "<Lane1C2>"
  Bus Selector/11 -> [Lane3_C2_Lane_Curvature]  "<Lane3C2>"
  Bus Selector/16 -> [Lane4_C3_Lane_Curvature_Driv]  "<Lane4C3>"
  Bus Selector/2 -> [Lane1_C1_Heading_Angle]  "<Lane1C1>"
  Bus Selector/5 -> [Lane2_C0_Lane_Position]  "<Lane2C0>"
  Bus Selector/13 -> [Lane4_C0_Lane_Position]  "<Lane4C0>"
  Bus Selector/9 -> [Lane3_C0_Lane_Position]  "<Lane3C0>"
  Bus Selector/6 -> [Lane2_C1_Heading_Angle]  "<Lane2C1>"
  [Lane3_Lane_Mark_Quality] -> Data Type Conversion45/1
  [Lane3_Lane_View_Range_Start] -> Data Type Conversion46/1
  [Lane3_Lane_View_Range_End] -> Data Type Conversion47/1
  [Lane3_C0_Lane_Position] -> Data Type Conversion48/1
  [Lane3_C1_Heading_Angle] -> Data Type Conversion55/1
  [Lane3_C2_Lane_Curvature] -> Data Type Conversion56/1
  [Lane3_C3_Lane_Curvature_Driv] -> Data Type Conversion57/1
  [Lane1_Lane_Mark_Quality] -> Data Type Conversion66/1
  [Lane1_Lane_View_Range_Start] -> Data Type Conversion67/1
  [Lane1_Lane_View_Range_End] -> Data Type Conversion68/1
  [Lane1_C0_Lane_Position] -> Data Type Conversion69/1
  [Lane1_C1_Heading_Angle] -> Data Type Conversion70/1
  [Lane1_C2_Lane_Curvature] -> Data Type Conversion71/1
  [Lane1_C3_Lane_Curvature_Driv] -> Data Type Conversion72/1
  Demux/2 -> Data Type Conversion85/1, [CCSwStsSetSwAHSC1_u8]
  Manual Switch/1 -> Demux/1
  Mux/1 -> Manual Switch/1
  Mux1/1 -> Manual Switch/2
  [OnSW] -> Mux1/1
  [SetSW] -> Mux1/2
  [SpdIncSW] -> Mux1/3
  [SpdDecSW] -> Mux1/4
  [RsmSW] -> Mux1/5
  [CanclSW] -> Mux1/6
  Constant5/1 -> Mux/6, Mux/5, Mux/4, Mux/3, Mux/2, Mux/1
  Constant6/1 -> Chart/6(CCCDuration)
  Mux2/1 -> V Compare/1
  Constant7/1 -> Chart/2(SteadyFlag)
  SetSpd/1 -> Chart/7(SetSpd)
  MemSpd/1 -> Chart/8(MemSpd)
  [SteadyFlag] -> Terminator_1/1
